simulink model "xpc_dlt_adept_ctf_204_c_m"  (R2013b)
settings: Solver=ode4  StartTime=0.0  StopTime=3.224  FixedStep=0.001  RelTol=1e-3
libraries: xpclib x6, xpcnilib x5, simulink x3
(part 1 of 2)
settings Model: BufferReuse=off  Creator=lucius  LastModifiedBy=lucius
settings OptimizationCC: BlockReduction=off  OptimizeBlockIOStorage=off  BufferReuse=off  ExpressionFolding=off  LocalBlockOutputs=off
settings HardwareCC: ProdIntDivRoundTo=Zero  ProdEndianess=LittleEndian  ProdHWDeviceType=Generic->32-bit x86 compatible
settings RTWCC: SystemTargetFile=xpctarget.tlc  TemplateMakefile=xpc_default_tmf  Description=xPC Target  ProcessScript=xpctarget_make_rtw_hook  RTWCompilerOptimization=On
settings xpcTargetCC: TargetFcnLib=ansi_tfl_table_tmw.mat  CodeReplacementLibrary=XPC_BLAS  ParMdlRefBuildCompliant=on  ConcurrentExecutionCompliant=on  CombineSignalStateStructs=off  MATLABClassNameForMDSCustomization=xpcAperiodicCustomization  GRTInterface=on  GenerateAllocFcn=off  xPCTaskExecutionProfile=off  xPCRL32EventNumber=5000  xPCLoadParamSetFile=off  xPCConcurrentTasks=off  xPCEnableSFAnimation=off

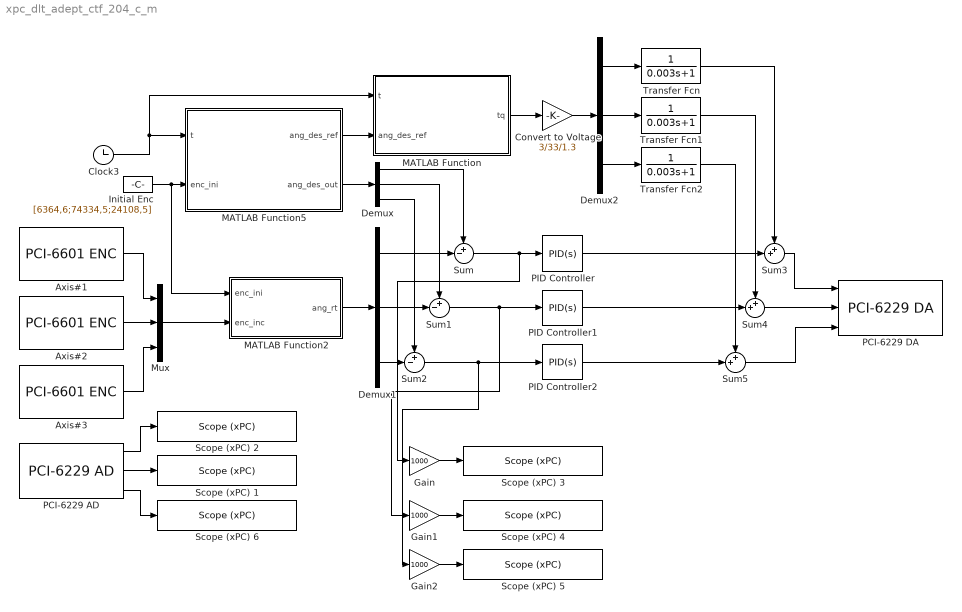
== system xpc_dlt_adept_ctf_204_c_m ==
  Axis#1 : xpcnilib/Incremental Encoder/PCI-6601 ENC  channel=1  countMode=Quadrature Mode X4  initCount=0  reload=off  indexPhase=A low B low  filter=None  sampleTime=0.001  slot=-1
  Axis#2 : xpcnilib/Incremental Encoder/PCI-6601 ENC  channel=2  countMode=Quadrature Mode X4  initCount=0  reload=off  indexPhase=A low B low  filter=None  sampleTime=0.001  slot=-1
  Axis#3 : xpcnilib/Incremental Encoder/PCI-6601 ENC  channel=3  countMode=Quadrature Mode X4  initCount=0  reload=off  indexPhase=A low B low  filter=None  sampleTime=0.001  slot=-1
  Clock3 : Clock
  Convert to Voltage : Gain  Gain=3/33/1.3
  Demux : Demux  Outputs=3
  Demux1 : Demux  Outputs=3
  Demux2 : Demux  Outputs=3
  Gain : Gain  Gain=1000
  Gain1 : Gain  Gain=1000
  Gain2 : Gain  Gain=1000
  Initial Enc : Constant  Value=[6364,6;74334,5;24108,5]
  MATLAB Function : MATLAB Function  TreatAsAtomicUnit=on
  MATLAB Function2 : MATLAB Function  TreatAsAtomicUnit=on
  MATLAB Function5 : MATLAB Function  TreatAsAtomicUnit=on
  Mux : Mux  Inputs=3
  PCI-6229 AD : xpcnilib/A//D/M Series/PCI-6229 AD  channel=[1,3,17]  range=[10]  coupling=[0]  scantime=5e-6  sampletime=0.001  slot=-1
  PCI-6229 DA : xpcnilib/D//A/M Series/PCI-6229 DA  channel=[1,2,3]  reset=[1,1,1]  initValue=[0,0,0]  sampletime=-1  slot=-1
  PID Controller : simulink/Continuous/PID Controller  Controller=PID  TimeDomain=Continuous-time  SampleTime=1  IntegratorMethod=Forward Euler  FilterMethod=Forward Euler  Form=Parallel  P=50  I=60  D=2  N=100  InitialConditionSource=internal  InitialConditionForIntegrator=0  InitialConditionForFilter=0  ExternalReset=none  LimitOutput=off  UpperSaturationLimit=inf  LowerSaturationLimit=-inf  LinearizeAsGain=on  AntiWindupMode=none  Kb=1  TrackingMode=off  Kt=1  PParamMin=[]  PParamMax=[]  IParamMin=[]  IParamMax=[]  DParamMin=[]  DParamMax=[]  NParamMin=[]  NParamMax=[]  KbParamMin=[]  KbParamMax=[]  KtParamMin=[]  KtParamMax=[]  POutMin=[]  POutMax=[]  IOutMin=[]  IOutMax=[]  DOutMin=[]  DOutMax=[]  NOutMin=[]  NOutMax=[]  KbOutMin=[]  KbOutMax=[]  KtOutMin=[]  KtOutMax=[]  IntegratorOutMin=[]  IntegratorOutMax=[]  FilterOutMin=[]  FilterOutMax=[]  SumOutMin=[]  SumOutMax=[]  SumI1OutMin=[]  SumI1OutMax=[]  SumI2OutMin=[]  SumI2OutMax=[]  SumI3OutMin=[]  SumI3OutMax=[]  SumDOutMin=[]  SumDOutMax=[]  SaturationOutMin=[]  SaturationOutMax=[]  IntegratorContinuousStateAttributes=''  IntegratorStateMustResolveToSignalObject=off  IntegratorRTWStateStorageClass=Auto  FilterContinuousStateAttributes=''  FilterStateMustResolveToSignalObject=off  FilterRTWStateStorageClass=Auto
  PID Controller1 : simulink/Continuous/PID Controller  Controller=PID  TimeDomain=Continuous-time  SampleTime=1  IntegratorMethod=Forward Euler  FilterMethod=Forward Euler  Form=Parallel  P=50  I=60  D=2  N=100  InitialConditionSource=internal  InitialConditionForIntegrator=0  InitialConditionForFilter=0  ExternalReset=none  LimitOutput=off  UpperSaturationLimit=inf  LowerSaturationLimit=-inf  LinearizeAsGain=on  AntiWindupMode=none  Kb=1  TrackingMode=off  Kt=1  PParamMin=[]  PParamMax=[]  IParamMin=[]  IParamMax=[]  DParamMin=[]  DParamMax=[]  NParamMin=[]  NParamMax=[]  KbParamMin=[]  KbParamMax=[]  KtParamMin=[]  KtParamMax=[]  POutMin=[]  POutMax=[]  IOutMin=[]  IOutMax=[]  DOutMin=[]  DOutMax=[]  NOutMin=[]  NOutMax=[]  KbOutMin=[]  KbOutMax=[]  KtOutMin=[]  KtOutMax=[]  IntegratorOutMin=[]  IntegratorOutMax=[]  FilterOutMin=[]  FilterOutMax=[]  SumOutMin=[]  SumOutMax=[]  SumI1OutMin=[]  SumI1OutMax=[]  SumI2OutMin=[]  SumI2OutMax=[]  SumI3OutMin=[]  SumI3OutMax=[]  SumDOutMin=[]  SumDOutMax=[]  SaturationOutMin=[]  SaturationOutMax=[]  IntegratorContinuousStateAttributes=''  IntegratorStateMustResolveToSignalObject=off  IntegratorRTWStateStorageClass=Auto  FilterContinuousStateAttributes=''  FilterStateMustResolveToSignalObject=off  FilterRTWStateStorageClass=Auto
  PID Controller2 : simulink/Continuous/PID Controller  Controller=PID  TimeDomain=Continuous-time  SampleTime=1  IntegratorMethod=Forward Euler  FilterMethod=Forward Euler  Form=Parallel  P=50  I=60  D=2  N=100  InitialConditionSource=internal  InitialConditionForIntegrator=0  InitialConditionForFilter=0  ExternalReset=none  LimitOutput=off  UpperSaturationLimit=inf  LowerSaturationLimit=-inf  LinearizeAsGain=on  AntiWindupMode=none  Kb=1  TrackingMode=off  Kt=1  PParamMin=[]  PParamMax=[]  IParamMin=[]  IParamMax=[]  DParamMin=[]  DParamMax=[]  NParamMin=[]  NParamMax=[]  KbParamMin=[]  KbParamMax=[]  KtParamMin=[]  KtParamMax=[]  POutMin=[]  POutMax=[]  IOutMin=[]  IOutMax=[]  DOutMin=[]  DOutMax=[]  NOutMin=[]  NOutMax=[]  KbOutMin=[]  KbOutMax=[]  KtOutMin=[]  KtOutMax=[]  IntegratorOutMin=[]  IntegratorOutMax=[]  FilterOutMin=[]  FilterOutMax=[]  SumOutMin=[]  SumOutMax=[]  SumI1OutMin=[]  SumI1OutMax=[]  SumI2OutMin=[]  SumI2OutMax=[]  SumI3OutMin=[]  SumI3OutMax=[]  SumDOutMin=[]  SumDOutMax=[]  SaturationOutMin=[]  SaturationOutMax=[]  IntegratorContinuousStateAttributes=''  IntegratorStateMustResolveToSignalObject=off  IntegratorRTWStateStorageClass=Auto  FilterContinuousStateAttributes=''  FilterStateMustResolveToSignalObject=off  FilterRTWStateStorageClass=Auto
  Scope (xPC) 1 : xpclib/Misc./Scope (xPC)   scopeno=2  scopetype=File  autostart=on  viewmode=Graphical redraw  formatstr='%15.6f'  grid=on  ylimits=[0,0]  nosamples=3224  noprepostsamples=0  interleave=1  triggermode=FreeRun  triggersignal=1  trigsignalfromport=off  triggerlevel=0.0  triggerslope=Either  triggerscope=1  triggersample=0  filename=a2t9fmc2.dat  mode=Lazy  writesize=512  autorestart=off  dynamicfilemode=off  maxwritefilesize=512*1024^2
  Scope (xPC) 2 : xpclib/Misc./Scope (xPC)   scopeno=1  scopetype=File  autostart=on  viewmode=Graphical redraw  formatstr='%15.6f'  grid=on  ylimits=[0,0]  nosamples=3224  noprepostsamples=0  interleave=1  triggermode=FreeRun  triggersignal=1  trigsignalfromport=off  triggerlevel=0.0  triggerslope=Either  triggerscope=1  triggersample=0  filename=a1t9fmc2.dat  mode=Lazy  writesize=512  autorestart=off  dynamicfilemode=off  maxwritefilesize=512*1024^2
  Scope (xPC) 3 : xpclib/Misc./Scope (xPC)   scopeno=4  scopetype=File  autostart=on  viewmode=Graphical redraw  formatstr='%15.6f'  grid=on  ylimits=[0,0]  nosamples=3224  noprepostsamples=0  interleave=1  triggermode=FreeRun  triggersignal=1  trigsignalfromport=off  triggerlevel=0.0  triggerslope=Either  triggerscope=1  triggersample=0  filename=a1e9fmc2.dat  mode=Lazy  writesize=512  autorestart=off  dynamicfilemode=off  maxwritefilesize=512*1024^2
  Scope (xPC) 4 : xpclib/Misc./Scope (xPC)   scopeno=5  scopetype=File  autostart=on  viewmode=Graphical redraw  formatstr='%15.6f'  grid=on  ylimits=[0,0]  nosamples=3224  noprepostsamples=0  interleave=1  triggermode=FreeRun  triggersignal=1  trigsignalfromport=off  triggerlevel=0.0  triggerslope=Either  triggerscope=1  triggersample=0  filename=a2e9fmc2.dat  mode=Lazy  writesize=512  autorestart=off  dynamicfilemode=off  maxwritefilesize=512*1024^2
  Scope (xPC) 5 : xpclib/Misc./Scope (xPC)   scopeno=6  scopetype=File  autostart=on  viewmode=Graphical redraw  formatstr='%15.6f'  grid=on  ylimits=[0,0]  nosamples=3224  noprepostsamples=0  interleave=1  triggermode=FreeRun  triggersignal=1  trigsignalfromport=off  triggerlevel=0.0  triggerslope=Either  triggerscope=1  triggersample=0  filename=a3e9fmc2.dat  mode=Lazy  writesize=512  autorestart=off  dynamicfilemode=off  maxwritefilesize=512*1024^2
  Scope (xPC) 6 : xpclib/Misc./Scope (xPC)   scopeno=3  scopetype=File  autostart=on  viewmode=Graphical redraw  formatstr='%15.6f'  grid=on  ylimits=[0,0]  nosamples=3224  noprepostsamples=0  interleave=1  triggermode=FreeRun  triggersignal=1  trigsignalfromport=off  triggerlevel=0.0  triggerslope=Either  triggerscope=1  triggersample=0  filename=a3t9fmc2.dat  mode=Lazy  writesize=512  autorestart=off  dynamicfilemode=off  maxwritefilesize=512*1024^2
  Sum : Sum  Inputs=+-|
  Sum1 : Sum  Inputs=+-|
  Sum2 : Sum  Inputs=+-|
  Sum3 : Sum  Inputs=++|
  Sum4 : Sum  Inputs=++|
  Sum5 : Sum  Inputs=++|
  Transfer Fcn : TransferFcn  Denominator=[0.003 1]
  Transfer Fcn1 : TransferFcn  Denominator=[0.003 1]
  Transfer Fcn2 : TransferFcn  Denominator=[0.003 1]
  wires:
  Demux/1 -> Sum/1
  Demux/3 -> Sum2/1
  Demux/2 -> Sum1/1
  Sum/1 -> Gain/1, PID Controller/1
  Sum1/1 -> Gain1/1, PID Controller1/1
  Sum2/1 -> Gain2/1, PID Controller2/1
  Axis#1/1 -> Mux/1
  Axis#2/1 -> Mux/2
  Axis#3/1 -> Mux/3
  MATLAB Function2/1(ang_rt) -> Demux1/1
  Demux1/1 -> Sum/2
  Demux1/2 -> Sum1/2
  Demux1/3 -> Sum2/2
  MATLAB Function5/2(ang_des_out) -> Demux/1
  Mux/1 -> MATLAB Function2/2(enc_inc)
  Initial Enc/1 -> MATLAB Function5/2(enc_ini), MATLAB Function2/1(enc_ini)
  Clock3/1 -> MATLAB Function5/1(t), MATLAB Function/1(t)
  MATLAB Function5/1(ang_des_ref) -> MATLAB Function/2(ang_des_ref)
  PID Controller/1 -> Sum3/2
  PID Controller2/1 -> Sum5/2
  PID Controller1/1 -> Sum4/2
  Sum3/1 -> PCI-6229 DA/1
  Sum4/1 -> PCI-6229 DA/2
  Sum5/1 -> PCI-6229 DA/3
  MATLAB Function/1(tq) -> Convert to Voltage/1
  Convert to Voltage/1 -> Demux2/1
  Gain/1 -> Scope (xPC) 3/1
  Gain1/1 -> Scope (xPC) 4/1
  Gain2/1 -> Scope (xPC) 5/1
  PCI-6229 AD/2 -> Scope (xPC) 1/1
  PCI-6229 AD/1 -> Scope (xPC) 2/1
  PCI-6229 AD/3 -> Scope (xPC) 6/1
  Demux2/3 -> Transfer Fcn2/1
  Demux2/2 -> Transfer Fcn1/1
  Demux2/1 -> Transfer Fcn/1
  Transfer Fcn2/1 -> Sum5/1
  Transfer Fcn1/1 -> Sum4/1
  Transfer Fcn/1 -> Sum3/1

== matlab function xpc_dlt_adept_ctf_204_c_m/MATLAB Function2 ==
  data: enc_ini input; ang_rt output; enc_inc input
function ang_rt = inc2jo(enc_ini,enc_inc)
%***********************REFERENCE****************************************
%LIMIT&ABSOLUTE NUMBER
%Axis#      Limit   Absolute Position
%1          -45     14circles   +1784
%           100     0circles    +98713

%2          -45     13circles   +120485
%           100     0circles    +87782

%3          -45     13circles   +77696
%           100     0circles    +44275

%************************COMPUTATION**************************************
enc_rt=[0,0,0];
enc_rt(1)=enc_ini(1,2)*131072+enc_ini(1,1)+enc_inc(1)*131072/10000;%real time
enc_rt(2)=enc_ini(2,2)*131072+enc_ini(2,1)+enc_inc(2)*131072/10000;%encoder
enc_rt(3)=enc_ini(3,2)*131072+enc_ini(3,1)+enc_inc(3)*131072/10000;%value
ang_rt=[0;0;0];
%Axis#1
ang_rt(1)=(enc_rt(1)-98713)*pi*29/36/(14*131072+1784-98713)-5*pi/9;
%Axis#2
ang_rt(2)=(enc_rt(2)-87782)*pi*29/36/(13*131072+120485-87782)-5*pi/9;
%Axis#3
ang_rt(3)=(enc_rt(3)-44275)*pi*29/36/(13*131072+77696-44275)-5*pi/9;

== matlab function xpc_dlt_adept_ctf_204_c_m/MATLAB Function ==
  data: t input; tq output; ang_des_ref input
function tq = ctf(t,ang_des_ref)
T=2;
if t<T
    tq=[0;0;0];
else
    torq=dltsdy([ang_des_ref(1);ang_des_ref(2);ang_des_ref(3)],[ang_des_ref(4);ang_des_ref(5);ang_des_ref(6)],[ang_des_ref(7);ang_des_ref(8);ang_des_ref(9)],[ang_des_ref(10);ang_des_ref(11);ang_des_ref(12)]);
    tq=-[torq(1);torq(3);torq(2)];%convert to the real torq comand
end
